simulink model "Model3Mod"  (R2020a)
settings: Solver=ode15s  StartTime=0.0  StopTime=200  RelTol=1e-3
values from neighbouring files (symbols this model uses):
  longStraight = 1006    [plotTrack.m]
  shortStraight = 201    [plotTrack.m]
  turn = 402    [plotTrack.m]
undefined symbols (not defined in the file or in its folder): a, a0, a1, a10, a11, a12, a13, a14, a15, a16, a17, a2, a3, a4, a5, a6, a7, a8, a9, Area, b, b1, b11, b12, b2, banking_indy, bankingON, C_fuel, camber, curveCenters, Cx, Cz, errorThreshold, g, init_x_pos, init_y_pos, init_yaw, IT, K_wear, l_f, l_r, lookahead, m_fuel, mT, rho_0, trajec, TyreContactAreaFront, TyreContactAreaRear, w1, w2
libraries: simulink x4, drivingvehiclecontroller x1
(part 2 of 2)

== matlab function Model3Mod/prova ==
  data: egox input; egoy input; curveCenters input; curvature output; trajec input
function curvature = curv(egox, egoy, curveCenters, trajec)

distArray = (egox - trajec(2,:)).^2 + (egoy - trajec(3,:)).^2;
% [min_dist, real_index] = min(distArray);
[~, real_index] = min(distArray);
% min_dist = sqrt(min_dist);

% long straight 1
if egoy < curveCenters(1,2) && egox >= curveCenters(4,1) && egox <= curveCenters(1,1)
    curvature = 0;
% long straight 2
elseif egoy > curveCenters(2,2) && egox >= curveCenters(4,1) && egox <= curveCenters(1,1)
    curvature = 0;
% short straigt 1
elseif egox > 0 && egoy >= curveCenters(1,2) && egoy <= curveCenters(2,2)
    curvature = 0;
% short straigt 2
elseif egox < 0 && egoy >= curveCenters(1,2) && egoy <= curveCenters(2,2)
    curvature = 0;
% curve 1
elseif egox > curveCenters(1,1) && egoy < curveCenters(1,2)
    Rcurv = pdist2([trajec(2,real_index), trajec(3, real_index)],curveCenters(1,:));
    curvature = 1/Rcurv;
% curve 2
elseif egox > curveCenters(2,1) && egoy > curveCenters(2,2)
    Rcurv = pdist2([trajec(2,real_index), trajec(3, real_index)],curveCenters(2,:));
    curvature = 1/Rcurv;
% curve 3
elseif egox < curveCenters(3,1) && egoy > curveCenters(3,2)
    Rcurv = pdist2([trajec(2,real_index), trajec(3, real_index)],curveCenters(3,:));
    curvature = 1/Rcurv;
% curve 4
elseif egox < curveCenters(4,1) && egoy < curveCenters(4,2)
    Rcurv = pdist2([trajec(2,real_index), trajec(3, real_index)],curveCenters(4,:));
    curvature = 1/Rcurv;
% default else
else
    curvature = 0;
end

== matlab function Model3Mod/DynamicModel1/lateral_error ==
  data: egox input; egoy input; trajec input; ref output; cur_yaw input; index output; lookAhead input; errorThreshold input
function [ref,index] = lateral_error(egox, egoy, trajec, cur_yaw, lookAhead, errorThreshold)%, curveCenters)

newEgox = egox + lookAhead*cos(cur_yaw);
newEgoy = egoy + lookAhead*sin(cur_yaw);

distArray = (newEgox - trajec(2,:)).^2 + (newEgoy - trajec(3,:)).^2;
[min_dist, real_index] = min(distArray);

min_dist = sqrt(min_dist);
index = real_index;

v1 = [newEgox - egox, newEgoy - egoy, 0];
v2 = [trajec(2, real_index) - egox, trajec(3, real_index) - egoy, 0];
C = cross(v1, v2);
if abs(C(3)) < errorThreshold
    ref = 0;
elseif sign(C(3)) == 1
    ref = -min_dist;
elseif sign(C(3)) == -1
    ref = min_dist;
else
    ref = 0;
end

% % long straight 1
% if newEgoy < curveCenters(1,2) && newEgox >= curveCenters(4,1) && newEgox <= curveCenters(1,1)
%     if newEgoy > -6.75 + threshold
%         ref = min_dist;
%     elseif newEgoy < -6.75 - threshold
%         ref = -min_dist;
%     else
%         ref = 0;
%     end
% % long straight 2
% elseif newEgoy > curveCenters(2,2) && newEgox >= curveCenters(4,1) && newEgox <= curveCenters(1,1)
%     if newEgoy < 720.04 - threshold
%         ref = min_dist;
%     elseif newEgoy > 720.04 + threshold
%         ref = -min_dist;
%     else
%         ref = 0;
%     end
% % short straigt 1
% elseif newEgox > 0 && newEgoy >= curveCenters(1,2) && newEgoy <= curveCenters(2,2)
%     if newEgox < 765.89 - threshold
%         ref = min_dist;
%     elseif newEgox > 765.89 + threshold
%         ref = -min_dist;
%     else
%         ref = 0;
%     end
% % short straigt 2
% elseif newEgox < 0 && newEgoy >= curveCenters(1,2) && newEgoy <= curveCenters(2,2)
%     if newEgox > -765.89 + threshold
%         ref = min_dist;
%     elseif newEgox < -765.89 - threshold
%         ref = -min_dist;
%     else
%         ref = 0;
%     end
% % curve 1
% elseif newEgox > curveCenters(1,1) && newEgoy < curveCenters(1,2)
%     myR = pdist2([newEgox,newEgoy],curveCenters(1,:));
%     trajR = pdist2([trajec(2, real_index),trajec(3, real_index)],curveCenters(1,:));
%     if myR > trajR + threshold
%         ref = -min_dist;
%     elseif myR < trajR - threshold
%         ref = min_dist;
%     else
%         ref = 0;
%     end
% % curve 2
% elseif newEgox > curveCenters(2,1) && newEgoy > curveCenters(2,2)
%     myR = pdist2([newEgox,newEgoy],curveCenters(2,:));
%     trajR = pdist2([trajec(2, real_index),trajec(3, real_index)],curveCenters(2,:));
%     if myR > trajR + threshold
%         ref = -min_dist;
%     elseif myR < trajR - threshold
%         ref = min_dist;
%     else
%         ref = 0;
%     end
% % curve 3
% elseif newEgox < curveCenters(3,1) && newEgoy > curveCenters(3,2)
%     myR = pdist2([newEgox,newEgoy],curveCenters(3,:));
%     trajR = pdist2([trajec(2, real_index),trajec(3, real_index)],curveCenters(3,:));
%     if myR > trajR + threshold
%         ref = -min_dist;
%     elseif myR < trajR - threshold
%         ref = min_dist;
%     else
%         ref = 0;
%     end
% % curve 4
% elseif newEgox < curveCenters(4,1) && newEgoy < curveCenters(4,2)
%     myR = pdist2([newEgox,newEgoy],curveCenters(4,:));
%     trajR = pdist2([trajec(2, real_index),trajec(3, real_index)],curveCenters(4,:));
%     if myR > trajR + threshold
%         ref = -min_dist;
%     elseif myR < trajR - threshold
%         ref = min_dist;
%     else
%         ref = 0;
%     end
% % default else
% else
%     ref = 0;
% end

== matlab function Model3Mod/DynamicModel1/Banking ==
  data: x input; res output; y input; curveCenters input; longStraight input; shortStraight input; curve input; bankingON input; banking_indy input
function res = calculateBanking(x, y, curveCenters, ...
    longStraight, shortStraight, curve, ...
    bankingON, banking_indy)

% coder.extrinsic('evalin')
% coder.extrinsic('fitresult')
% fun = evalin('base','fitresult');

init_x = -271.4;
totL = 4023.4;
initD = pdist2([init_x, 0], [curveCenters(1,1),0]);

R = curve * 2 / pi;


if (bankingON < 1)
    res = 0;
else
    % long straight 1
    if y < curveCenters(1,2) && x >= curveCenters(4,1) && x <= curveCenters(1,1)
        d = pdist2([x, 0],[init_x, 0]);
        l = (totL - d)*(x < init_x) + ...
            (d)*(x >= init_x);
    % long straight 2
    elseif y > curveCenters(2,2) && x >= curveCenters(4,1) && x <= curveCenters(1,1)
        d = pdist2([x, 0],[curveCenters(2,1),0]);
        l = d + initD + shortStraight + 2*curve;
    % short straigt 1
    elseif x > 0 && y >= curveCenters(1,2) && y <= curveCenters(2,2)
        d = pdist2([y, 0],[curveCenters(1,2),0]);
        l = d + initD + curve;
    % short straigt 2
    elseif x < 0 && y >= curveCenters(1,2) && y <= curveCenters(2,2)
        d = pdist2([y, 0],[curveCenters(3,2),0]);
        l = d + initD + longStraight + shortStraight + 3*curve;
    % curve 1
    elseif x > curveCenters(1,1) && y < curveCenters(1,2)
        ang = asin((x - curveCenters(1,1))/pdist2([x,y],curveCenters(1,:)));
        l = ang * R + initD;
    % curve 2
    elseif x > curveCenters(2,1) && y > curveCenters(2,2)
        ang = asin((y - curveCenters(2,2))/pdist2([x,y],curveCenters(2,:)));
        l = ang * R + initD + curve + shortStraight;
    % curve 3
    elseif x < curveCenters(3,1) && y > curveCenters(3,2)
        ang = asin((-x + curveCenters(3,1))/pdist2([x,y],curveCenters(3,:)));
        l = ang * R + initD + curve*2 + shortStraight + longStraight;
    % curve 4
    elseif x < curveCenters(4,1) && y < curveCenters(4,2)
        ang = asin((-y + curveCenters(4,2))/pdist2([x,y],curveCenters(4,:)));
        l = ang * R + initD + curve*3 + shortStraight*2 + longStraight;
    % default else
    else 
        l = 0;
    end
    
    %res = fun(l);
    res = banking_indy(ceil(l*10),1);
    %res = 0;
end

% function res = calculateBanking(x, y, curveCenters, ...
%     bankingThresholdLong, bankingThresholdShort, bankingAngle, midY, ...
%     bankingON)
% if (bankingON < 1)
%     res = 0;
% else
%     if(y < curveCenters(1,2) || y > curveCenters(2,2)) 
%        if(abs(x) < curveCenters(1,1) - bankingThresholdLong)
%            res = 0;
%        elseif (abs(x) > curveCenters(1,1))
%            res = bankingAngle;
%        else
%            res = bankingAngle*( 1 - ((abs(x) -  curveCenters(1,1))/(-bankingThresholdLong)) );
%        end
%     else
%         if (abs(y-midY) < curveCenters(2,2) - bankingThresholdShort - midY)
%             res = 0;
%         else
%             res = bankingAngle*( 1 - ((abs(y-midY) -  curveCenters(2,2) + midY)/(-bankingThresholdShort)) );
%         end
%     end
% end

== matlab function Model3Mod/periodic ==
  data: yaw input; periodicYaw output
function periodicYaw = periodic(yaw)

periodicYaw = abs(yaw) - (2*pi * floor(abs(yaw)/(2*pi)));

== matlab function Model3Mod/DynamicModel1/periodic ==
  data: yaw input; periodicYaw output
function periodicYaw = periodic(yaw)

periodicYaw = abs(yaw) - (2*pi * floor(abs(yaw)/(2*pi)));

== matlab function Model3Mod/prova1 ==
  data: xref output; yref output; yaw_ref output; egox input; egoy input; curveCenters input; curvature output; trajec input; error output
function [xref, yref, yaw_ref, curvature, error] = curv(egox, egoy, curveCenters, trajec)

distArray = (egox - trajec(2,:)).^2 + (egoy - trajec(3,:)).^2;
% [min_dist, real_index] = min(distArray);
[error, real_index] = min(distArray);
xref = trajec(2, real_index);
yref = trajec(3, real_index);
yaw_ref = trajec(4, real_index);
error = sqrt(error);

% long straight 1
if egoy < curveCenters(1,2) && egox >= curveCenters(4,1) && egox <= curveCenters(1,1)
    curvature = 0;
% long straight 2
elseif egoy > curveCenters(2,2) && egox >= curveCenters(4,1) && egox <= curveCenters(1,1)
    curvature = 0;
% short straigt 1
elseif egox > 0 && egoy >= curveCenters(1,2) && egoy <= curveCenters(2,2)
    curvature = 0;
% short straigt 2
elseif egox < 0 && egoy >= curveCenters(1,2) && egoy <= curveCenters(2,2)
    curvature = 0;
% curve 1
elseif egox > curveCenters(1,1) && egoy < curveCenters(1,2)
    Rcurv = pdist2([trajec(2,real_index), trajec(3, real_index)],curveCenters(1,:));
    curvature = 1/Rcurv;
% curve 2
elseif egox > curveCenters(2,1) && egoy > curveCenters(2,2)
    Rcurv = pdist2([trajec(2,real_index), trajec(3, real_index)],curveCenters(2,:));
    curvature = 1/Rcurv;
% curve 3
elseif egox < curveCenters(3,1) && egoy > curveCenters(3,2)
    Rcurv = pdist2([trajec(2,real_index), trajec(3, real_index)],curveCenters(3,:));
    curvature = 1/Rcurv;
% curve 4
elseif egox < curveCenters(4,1) && egoy < curveCenters(4,2)
    Rcurv = pdist2([trajec(2,real_index), trajec(3, real_index)],curveCenters(4,:));
    curvature = 1/Rcurv;
% default else
else
    curvature = 0;
end
